simulink model "power_3phlinereclose"  (Simulink 6.0)
settings: Solver=FixedStepDiscrete  StartTime=0.0  StopTime=0.7  FixedStep=50e-6  RelTol=1e-4
undefined symbols (not defined in the file or in its folder): D1, Delta, rvar
libraries: powerlib x24, powerlib_extras x2
settings Model: Creator=sybille  LastModifiedBy=batserve  ExtModeTrigMode=oneshot  ExtModeArmWhenConnect=off  ExtModeAutoUpdateStatusClock=off
settings DataIOCC: LimitDataPoints=off  SignalLoggingName=sigsOut
settings OptimizationCC: BlockReduction=off  BooleanDataType=off
settings DebuggingCC: CheckExecutionContextPreStartOutputMsg=on  CheckExecutionContextRuntimeOutputMsg=on  SolverPrmCheckMsg=none
settings HardwareCC: TargetUnknown=on

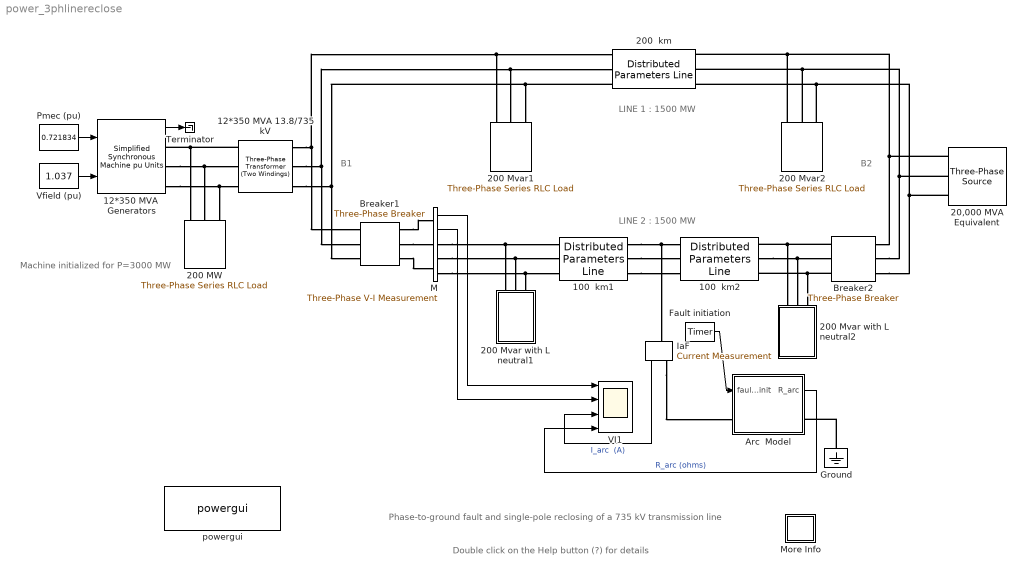
== system power_3phlinereclose ==
  note: Machine initialized
      |  for P=3000 MW
  note: Phase-to-ground fault and single-pole reclosing
      | of  a 735 kV transmission line
  note: Double click on the Help button (?) for details
  note: LINE 1 : 1500 MW
  note: LINE 2 : 1500 MW
  note: B1
  note: B2
  " Breaker1" : powerlib/Elements/Three-Phase Breaker  InitialState=closed  SwitchA=on  SwitchB=off  SwitchC=off  SwitchTimes="[4/60  34/60]"  External=off  BreakerResistance=0.001  SnubberResistance=1e5  SnubberCapacitance=inf  Measurements=None
      settings: AttributesFormatString=\n
  " Breaker2" : powerlib/Elements/Three-Phase Breaker  InitialState=closed  SwitchA=on  SwitchB=off  SwitchC=off  SwitchTimes="[4/60  34/60]"  External=off  BreakerResistance=0.001  SnubberResistance=1e5  SnubberCapacitance=inf  Measurements=None
      settings: AttributesFormatString=\n
  100  km1 : powerlib/Elements/Distributed Parameters Line  Phases=3  Frequency=60  Resistance=[0.01165 0.2676]  Inductance="[0.8679e-3  3.008e-3]"  Capacitance="[13.41e-9  8.57e-9]"  Length=100  x1=[0 4.02705178345773e-008 472803.943791492 -555536.540470784;0.000101545182061977 3.40498179648926e-008 493719.170547751 -537034.187151238;0.000203090364123953 2.77792247481943e-008 513910.94844655 -517744.915291176;0.00030463554618593 2.14679265121164e-008 533349.690387524 -497696.989544924;0.000406180728247907 1.51251712295358e-008 552006.912697188 -476919.786225657;0.000507725910309884 8.76025296747684e-009 569855.276866184 -455443.750260167]  x2=[0 2.22321217810247e-008 426110.546159933 -596874.196271499;0.000101545182061977 1.8422129253629e-008 448642.075203804 -580128.633772847;0.000203090364123953 1.45851426997592e-008 470516.207054946 -562533.006252784;0.00030463554618593 1.0726784472575e-008 491700.889452397 -544113.096661183;0.000406180728247907 6.8527082412422e-009 512165.080388495 -524895.895772037;0.000507725910309884 2.96859070658684e-009 531878.79359486 -504909.562633762]  x3=[0 -4.58387424712223e-010 398.802996869194 -914.417744018894;0.000101545182061977 -4.6900146555621e-010 433.507996432241 -898.484331192913;0.000203090364123953 -4.78928276503843e-010 467.577774834296 -881.234365351327;0.00030463554618593 -4.88153311755674e-010 500.962409480231 -862.69312294444;0.000406180728247907 -4.96663053827248e-010 533.612981719056 -842.88777253575;0.000507725910309884 -5.04445033356331e-010 565.481648524631 -821.847334991732]  x4=[0 5.9976805423792e-010 2831.47677973377 -3826.92877538475;0.000101545182061977 5.94374114547943e-010 2975.86707537689 -3715.75790695924;0.000203090364123953 5.88109235871343e-010 3115.89681999411 -3599.14232224004;0.00030463554618593 5.80982598162212e-010 3251.36082738892 -3477.25289855288;0.000406180728247907 5.73004644113919e-010 3382.06060155949 -3350.26824100279;0.000507725910309884 5.64187063857384e-010 3507.80462755576 -3218.3744207632]  x5=0.000507725910309884  Measurements=None
      settings: AttributesFormatString=\n
  100  km2 : powerlib/Elements/Distributed Parameters Line  Phases=3  Frequency=60  Resistance=[0.01165 0.2676]  Inductance="[0.8679e-3  3.008e-3]"  Capacitance="[13.41e-9  8.57e-9]"  Length=100  x1=[0 2.22321217810247e-008 426110.546159933 -596874.196271499;0.000101545182061977 1.8422129253629e-008 448642.075203804 -580128.633772847;0.000203090364123953 1.45851426997592e-008 470516.207054946 -562533.006252784;0.00030463554618593 1.0726784472575e-008 491700.889452397 -544113.096661183;0.000406180728247907 6.8527082412422e-009 512165.080388495 -524895.895772037;0.000507725910309884 2.96859070658684e-009 531878.79359486 -504909.562633762]  x2=[0 4.59735852839934e-009 372729.13846345 -628102.297137415;0.000101545182061977 3.36982514336241e-009 396494.954357377 -613376.898276943;0.000203090364123953 2.13735393882152e-009 419679.784462561 -597752.715567833;0.00030463554618593 9.01750860216852e-010 442249.655946163 -581252.643193266;0.000406180728247907 -3.3517355786267e-010 464171.497076899 -563900.858781373;0.000507725910309884 -1.57160684466362e-009 485413.185685194 -545722.787977656]  x3=[0 -5.35956762016625e-010 506.939672451892 -849.356884933018;0.000101545182061977 -5.42195113669513e-010 539.075463597358 -829.332546268725;0.000203090364123953 -5.47638984453713e-010 570.421345111015 -808.09298300137;0.00030463554618593 -5.52280397441583e-010 600.931385735744 -785.669317555797;0.000406180728247907 -5.56112551550395e-010 630.560878975732 -762.094407426942;0.000507725910309884 -5.59129831507993e-010 659.266408605095 -737.402797033607]  x4=[0 5.99099720181025e-010 2312.99164112511 -4150.97769376106;0.000101545182061977 5.97237056827686e-010 2470.16390621821 -4059.41308469481;0.000203090364123953 5.94499259405894e-010 2623.71662934839 -3961.90019990165;0.00030463554618593 5.90890339622171e-010 2773.42480903965 -3858.58192543766;0.000406180728247907 5.86415585642443e-010 2919.06907724226 -3749.60965402176;0.000507725910309884 5.81081554343263e-010 3060.43602077378 -3635.14306319931]  x5=0.000507725910309884  Measurements=None
      settings: AttributesFormatString=\n
  12*350 MVA 13.8/735 kV : powerlib/Elements/Three-Phase Transformer (Two Windings)  NominalPower=[ 12*350e6 , 60 ]  Winding1Connection=Delta (D1)  Winding1=[ 13.8e3 , 0.002 , 0.08 ]  Winding2Connection=Yg  Winding2=[ 735e3 , 0.002 , 0.08 ]  SetSaturation=off  Rm=500  Lm=500  Saturation=[ 0,0 ; 0.0024,1.2 ; 1.0,1.52 ]  Hysteresis=off  DataFile='hysteresis'  SetInitialFlux=off  InitialFluxes=[ 0.8 , -0.8 , 0.7 ]  Measurements=None  TransfoNumber=0
  12*350 MVA  Generators : powerlib/Machines/Simplified Synchronous Machine pu Units  ConnectionType=3-wire Y  NominalParameters=[ 12*350e6,13.8e3,60 ]  Mechanical=[ inf,0,2 ]  InternalRL=[ 0.22/15, 0.22 ]  InitialConditions=[0 2.57592 0.717405 0.717405 0.717405 -11.4303 -131.43 108.57]  Units=0  LoadFlowParameters=[1 3000000000 0 0 0]
      settings: AttributesFormatString=\n
  20,000 MVA Equivalent : powerlib/Electrical Sources/Three-Phase Source  Orientation=left  Voltage=735e3  PhaseAngle=0  Frequency=60  InternalConnection=Yg  SpecifyImpedance=on  Resistance=735^2/20000/10  Inductance=735^2/20000/377  ShortCircuitLevel=20000e6  BaseVoltage=735e3  XRratio=10
  200  km : powerlib/Elements/Distributed Parameters Line  Phases=3  Frequency=60  Resistance=[0.01165 0.2676]  Inductance="[0.8679e-3  3.008e-3]"  Capacitance="[13.41e-9  8.57e-9]"  Length=200  x1=[0 7.02850624185661e-008 397648.481541654 -611590.683160231;0.000203090364123953 5.84450393918789e-008 443263.140154233 -579383.379701848;0.000406180728247907 4.62625827673498e-008 486280.688841777 -543781.428257846;0.00060927109237186 3.38090704154687e-008 526449.08475992 -504993.423166597;0.000812361456495814 2.11574683413028e-008 563532.978450831 -463246.626078958;0.00101545182061977 8.38190317153931e-009 597315.092772245 -418785.634416262]  x2=[0 1.07284970616671e-008 289091.132559122 -670718.411670409;0.000203090364123953 8.34931711874698e-009 339546.435190599 -646641.332353954;0.000406180728247907 5.92121793939131e-009 388012.311368668 -618775.53597519;0.00060927109237186 3.45842592752685e-009 434204.796114864 -587284.290195669;0.000812361456495814 9.75370754826919e-010 477853.244411074 -552352.104440056;0.00101545182061977 -1.51339918375015e-009 518701.916927735 -514183.648842435]  x3=[0 -3.94575629964779e-010 275.972756440155 -952.973890092729;0.000203090364123953 -4.20081661821716e-010 348.056371840659 -929.072582426811;0.000406180728247907 -4.43126405666159e-010 418.100700470185 -899.727773133261;0.00060927109237186 -4.63574840722552e-010 485.69534767915 -865.111395514356;0.000812361456495814 -4.81307158171201e-010 550.444271673768 -825.426269362086;0.00101545182061977 -4.96219463116572e-010 611.968103952785 -780.904912622723]  x4=[0 5.79618896597322e-010 1755.99549575464 -4400.33732412217;0.000203090364123953 5.84376073526628e-010 2087.4253958724 -4253.13324126328;0.000406180728247907 5.85709349925921e-010 2406.62492372979 -4081.00975150415;0.00060927109237186 5.83610914034972e-010 2711.72386683501 -3884.97533848145;0.000812361456495814 5.78093060737307e-010 3000.93462901443 -3666.17858161356;0.00101545182061977 5.69188119523618e-010 3272.56270406429 -3425.90142649296]  x5=0.00101545182061977  Measurements=None
      settings: AttributesFormatString=\n
  200 MW : powerlib/Elements/Three-Phase Series RLC Load  Orientation=down  PhysicalDomain=powersysdomain  SubClassName=unknown  LeftPortType=p1  RightPortType=p1  LConnTagsString=A|B|C  Configuration=Y (grounded)  NominalVoltage=13.8e3  NominalFrequency=60  ActivePower=200e6  InductivePower=0  CapacitivePower=0  Measurements=None
  200 Mvar with L neutral1 : Subsystem  Orientation=down
  200 Mvar with L neutral2 : Subsystem  Orientation=down
  200 Mvar1 : powerlib/Elements/Three-Phase Series RLC Load  Orientation=down  PhysicalDomain=powersysdomain  SubClassName=unknown  LeftPortType=p1  RightPortType=p1  LConnTagsString=A|B|C  Configuration=Y (grounded)  NominalVoltage=735e3  NominalFrequency=60  ActivePower=200e6/250  InductivePower=200e6  CapacitivePower=0  Measurements=None
  200 Mvar2 : powerlib/Elements/Three-Phase Series RLC Load  Orientation=down  PhysicalDomain=powersysdomain  SubClassName=unknown  LeftPortType=p1  RightPortType=p1  LConnTagsString=A|B|C  Configuration=Y (grounded)  NominalVoltage=735e3  NominalFrequency=60  ActivePower=200e6/250  InductivePower=200e6  CapacitivePower=0  Measurements=None
  Arc  Model : Subsystem  mask(Arc model){Rarc_var=on, Rarc_fixed=0.1, Rparam=[56.54 0.006375], I0=50, Ts=50e-6}
      mask prompts: Rarc_var "Variable arc resistance :"; Rarc_fixed "Arc resistance for fixed arc resistance :"; Rparam "Arc parameters for variable arc resistance [Ro k] : :"; I0 "Current threshold for arc extinction Io (A rms) :"; Ts "Sample time (s) :"
      mask help:
      | This block implements a variable or fixed arc resistance model.
      |
      | Input 1, output 1:  Connection terminals of the arc
      |                              resistance.
      | Input 2 :    Control signal for the fault initiation
      | Use a short pulse of 1 cycle. Once fault current starts flowing, it is sustained by the arc ionized path.
      | Output 2:  Arc resitance
      |
      | If you check the 'Variable arc resistance' box, the mean arc resistance will be a function of the arc current, according to equation. Otherwise, the resistance will be kept constant.
      |
      |        Rarc= Ro*exp(-k*i)
      |
      | where:   i = rms value of the arc current (A)
      |              Ro, k = arc parameters
      |
      | The arc extinguishes at the next zero current crossing after its  rms value has fallen  below  the specified threshold current Io.
      mask init:
      | if strcmp(Rarc_var,'on'), rvar=1; else, rvar=0; end
      | R0=Rparam(1);
      | k=Rparam(2);
  Fault initiation : powerlib_extras/Control  Blocks/Timer  t=[ 1/60 2/60 ]  e="[1 0  ]"
  Ground : powerlib/Elements/Ground  Orientation=down  PhysicalDomain=powersysdomain  SubClassName=unknown  LeftPortType=p1  RightPortType=p1  LConnTagsString=a
  IaF : powerlib/Measurements/Current Measurement  Tag=PoWeRsYsTeMmEaSuReMeNt  Orientation=down  PhasorSimulation=off  OutputType=Magnitude  PSBequivalent=0
  M : powerlib/Measurements/Three-Phase V-I Measurement  VoltageMeasurement=phase-to-ground  SetLabelV=off  LabelV=V1  Vpu=on  Vbase=735e3  CurrentMeasurement=yes  SetLabelI=off  LabelI=I1  Ipu=on  Pbase=100e6  OutputType=Magnitude  PhasorSimulation=off  PSBequivalent=0
  More Info : Subsystem
      mask Display: disp('?')
  Pmec (pu) : Constant  Value=0.721834
  Terminator : Terminator
  VI1 : Scope  NumInputPorts=4
      settings: TimeRange=0.7000000000000001  YMin=-2~-100~-50000~0  YMax=2~100~50000~100  DataFormat=Array
  Vfield (pu) : Constant  Value=1.037
  powergui : powerlib/powergui  Priority=2  Frange=logspace(0,3,50)  Ylog=off  Xlog=off  save=off  variable=ZData  ZoomFFT=on  StartTime=0.0  cycles=1  DisplayStyle=off  fundamental=60  FreqAxis=off  MaxFrequency=1000  frequencyindice=60  frequencyindicesteady=1  RmsSteady=1  display=off  Ts=50e-6  methode=off  frequency=60  echomessages=on
  wires:
  Fault initiation/1 -> Arc  Model/1(fault_init)
  Arc  Model/1(R_arc) -> VI1/4  "R_arc (ohms)"
  Vfield (pu)/1 -> 12*350 MVA  Generators/2
  Pmec (pu)/1 -> 12*350 MVA  Generators/1
  M/1 -> VI1/1
  IaF/1 -> VI1/3  "I_arc  (A)"
  M/2 -> VI1/2
  12*350 MVA  Generators/1 -> Terminator/1
  connections:
  " Breaker1"/RConn1 -- M/LConn1
  " Breaker1"/RConn2 -- M/LConn2
  " Breaker1"/RConn3 -- M/LConn3
  " Breaker2"/LConn1 -- 100  km2/RConn1 -- 200 Mvar with L neutral2/LConn1
  100  km2/RConn2 -- " Breaker2"/LConn2 -- 200 Mvar with L neutral2/LConn2
  " Breaker2"/LConn3 -- 100  km2/RConn3 -- 200 Mvar with L neutral2/LConn3
  100  km1/RConn1 -- 100  km2/LConn1 -- IaF/LConn1
  " Breaker2"/RConn1 -- 200 Mvar2/LConn1 -- 200  km/RConn1 -- 20,000 MVA Equivalent/RConn1
  " Breaker2"/RConn2 -- 200 Mvar2/LConn2 -- 200  km/RConn2 -- 20,000 MVA Equivalent/RConn2
  " Breaker2"/RConn3 -- 200 Mvar2/LConn3 -- 200  km/RConn3 -- 20,000 MVA Equivalent/RConn3
  M/RConn1 -- 100  km1/LConn1 -- 200 Mvar with L neutral1/LConn1
  M/RConn2 -- 100  km1/LConn2 -- 200 Mvar with L neutral1/LConn2
  M/RConn3 -- 100  km1/LConn3 -- 200 Mvar with L neutral1/LConn3
  100  km1/RConn3 -- 100  km2/LConn3
  100  km1/RConn2 -- 100  km2/LConn2
  12*350 MVA  Generators/RConn2 -- 12*350 MVA 13.8/735 kV/LConn2 -- 200 MW/LConn2
  12*350 MVA 13.8/735 kV/LConn1 -- 12*350 MVA  Generators/RConn1 -- 200 MW/LConn1
  12*350 MVA  Generators/RConn3 -- 12*350 MVA 13.8/735 kV/LConn3 -- 200 MW/LConn3
  12*350 MVA 13.8/735 kV/RConn1 -- " Breaker1"/LConn1 -- 200  km/LConn1 -- 200 Mvar1/LConn1
  12*350 MVA 13.8/735 kV/RConn2 -- " Breaker1"/LConn2 -- 200  km/LConn2 -- 200 Mvar1/LConn2
  200  km/LConn3 -- 12*350 MVA 13.8/735 kV/RConn3 -- " Breaker1"/LConn3 -- 200 Mvar1/LConn3
  IaF/RConn1 -- Arc  Model/LConn1
  Ground/LConn1 -- Arc  Model/RConn1

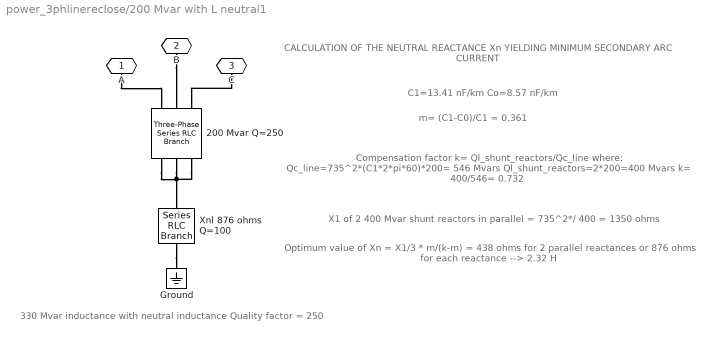
== system power_3phlinereclose/200 Mvar with L neutral1 ==
  note: CALCULATION OF THE NEUTRAL REACTANCE Xn
      | YIELDING MINIMUM SECONDARY ARC CURRENT
  note: X1 of 2 400 Mvar shunt reactors in parallel = 735^2*/ 400 = 1350 ohms
  note: Optimum value of Xn = X1/3 * m/(k-m) = 438 ohms for 2 parallel reactances
      | or 876 ohms for each reactance --> 2.32 H
  note: Compensation factor k= Ql_shunt_reactors/Qc_line
      | where:
      |  Qc_line=735^2*(C1*2*pi*60)*200= 546 Mvars
      |  Ql_shunt_reactors=2*200=400 Mvars
      | k= 400/546= 0.732
  note: m= (C1-C0)/C1 = 0.361
  note: C1=13.41 nF/km Co=8.57 nF/km
  note: 330 Mvar inductance
      | with neutral inductance
      | Quality factor = 250
  200 Mvar Q=250 : powerlib/Elements/Three-Phase Series RLC Branch  Orientation=down  PhysicalDomain=powersysdomain  SubClassName=unknown  LeftPortType=p1  RightPortType=p1  LConnTagsString=A|B|C  RConnTagsString=A|B|C  Resistance=735^2/200/250  Inductance=735^2/200/377  Capacitance=inf  Measurements=None
  Ground : powerlib/Elements/Ground  Orientation=down  PhysicalDomain=powersysdomain  SubClassName=unknown  LeftPortType=p1  RightPortType=p1  LConnTagsString=a
  Xnl 876 ohms Q=100 : powerlib/Elements/Series RLC Branch  Orientation=down  PhysicalDomain=powersysdomain  SubClassName=unknown  LeftPortType=p1  RightPortType=p1  LConnTagsString=__new0  RConnTagsString=__new0  Resistance=876/100  Inductance=876/377  Capacitance=inf  Measurements=None
  A : PMIOPort  Orientation=down  Port=1  Side=Left
  B : PMIOPort  Orientation=down  Port=2  Side=Left
  C : PMIOPort  Orientation=down  Port=3  Side=Left
  connections:
  A/RConn1 -- 200 Mvar Q=250/LConn1
  B/RConn1 -- 200 Mvar Q=250/LConn2
  C/RConn1 -- 200 Mvar Q=250/LConn3
  200 Mvar Q=250/RConn3 -- 200 Mvar Q=250/RConn2 -- Xnl 876 ohms Q=100/LConn1 -- 200 Mvar Q=250/RConn1
  Xnl 876 ohms Q=100/RConn1 -- Ground/LConn1

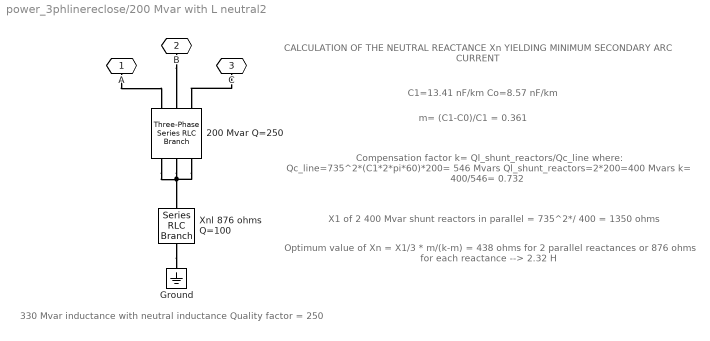
== system power_3phlinereclose/200 Mvar with L neutral2 ==
  note: 330 Mvar inductance
      | with neutral inductance
      | Quality factor = 250
  note: C1=13.41 nF/km Co=8.57 nF/km
  note: m= (C1-C0)/C1 = 0.361
  note: Compensation factor k= Ql_shunt_reactors/Qc_line
      | where:
      |  Qc_line=735^2*(C1*2*pi*60)*200= 546 Mvars
      |  Ql_shunt_reactors=2*200=400 Mvars
      | k= 400/546= 0.732
  note: Optimum value of Xn = X1/3 * m/(k-m) = 438 ohms for 2 parallel reactances
      | or 876 ohms for each reactance --> 2.32 H
  note: X1 of 2 400 Mvar shunt reactors in parallel = 735^2*/ 400 = 1350 ohms
  note: CALCULATION OF THE NEUTRAL REACTANCE Xn
      | YIELDING MINIMUM SECONDARY ARC CURRENT
  200 Mvar Q=250 : powerlib/Elements/Three-Phase Series RLC Branch  Orientation=down  PhysicalDomain=powersysdomain  SubClassName=unknown  LeftPortType=p1  RightPortType=p1  LConnTagsString=A|B|C  RConnTagsString=A|B|C  Resistance=735^2/200/250  Inductance=735^2/200/377  Capacitance=inf  Measurements=None
  Ground : powerlib/Elements/Ground  Orientation=down  PhysicalDomain=powersysdomain  SubClassName=unknown  LeftPortType=p1  RightPortType=p1  LConnTagsString=a
  Xnl 876 ohms Q=100 : powerlib/Elements/Series RLC Branch  Orientation=down  PhysicalDomain=powersysdomain  SubClassName=unknown  LeftPortType=p1  RightPortType=p1  LConnTagsString=__new0  RConnTagsString=__new0  Resistance=876/100  Inductance=876/377  Capacitance=inf  Measurements=None
  A : PMIOPort  Orientation=down  Port=1  Side=Left
  B : PMIOPort  Orientation=down  Port=2  Side=Left
  C : PMIOPort  Orientation=down  Port=3  Side=Left
  connections:
  Xnl 876 ohms Q=100/RConn1 -- Ground/LConn1
  200 Mvar Q=250/RConn3 -- 200 Mvar Q=250/RConn2 -- Xnl 876 ohms Q=100/LConn1 -- 200 Mvar Q=250/RConn1
  C/RConn1 -- 200 Mvar Q=250/LConn3
  B/RConn1 -- 200 Mvar Q=250/LConn2
  A/RConn1 -- 200 Mvar Q=250/LConn1

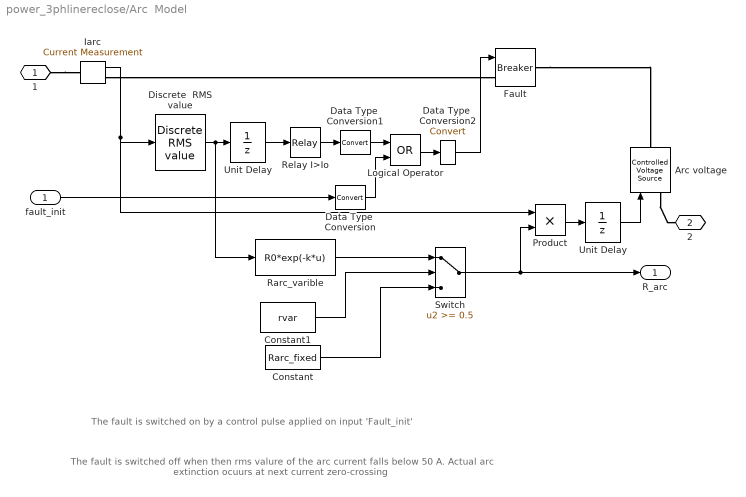
== system power_3phlinereclose/Arc  Model ==
  note: The fault is switched on by a control pulse applied on input 'Fault_init'
  note: The fault is switched off when then rms valure of the arc current falls below  50 A.
      | Actual arc extinction ocuurs at next current zero-crossing
  fault_init : Inport  Port=1  LatchInput=off
  Arc voltage : powerlib/Electrical Sources/Controlled Voltage Source  Description=source block  Orientation=up  Initialize=on  Amplitude=0  Phase=0  Frequency=0  Measurements=None
      settings: AttributesFormatString=\n
  Constant : Constant  Value=Rarc_fixed
  Constant1 : Constant  Value=rvar
  Data Type  Conversion : DataTypeConversion  OutDataTypeMode=boolean  SaturateOnIntegerOverflow=on  RndMeth=Zero
  Data Type  Conversion1 : DataTypeConversion  OutDataTypeMode=boolean  SaturateOnIntegerOverflow=on  RndMeth=Zero
  Data Type  Conversion2 : DataTypeConversion  OutDataTypeMode=double  SaturateOnIntegerOverflow=on  RndMeth=Zero
  Discrete  RMS value : powerlib_extras/Discrete Measurements/Discrete  RMS value  Freq=60  Mag_Init=0  Ts=Ts
  Fault : powerlib/Elements/Breaker  BreakerResistance=.001  InitialState=0  SnubberResistance=inf  SnubberCapacitance=0  SwitchingTimes="[ 4/60  5/60 ]"  External=on  Measurements=None
      settings: AttributesFormatString=\n
  Iarc : powerlib/Measurements/Current Measurement  Tag=PoWeRsYsTeMmEaSuReMeNt  PhasorSimulation=off  OutputType=Magnitude  PSBequivalent=0
  Logical Operator : Logic  Operator=OR
  Product : Product  SaturateOnIntegerOverflow=on  InputSameDT=on
  Rarc_varible : Fcn  Expr=R0*exp(-k*u)
  Relay I>Io : Relay  OnSwitchValue=I0*1.2  OffSwitchValue=I0  ZeroCross=off
  Switch : Switch  Threshold=0.5  ZeroCross=off  InputSameDT=on
  Unit Delay : UnitDelay  SampleTime=Ts
  "Unit Delay " : UnitDelay  SampleTime=Ts
  1 : PMIOPort  Port=1  Side=Left
  2 : PMIOPort  Orientation=left  Port=2  Side=Right
  R_arc : Outport
  wires:
  Discrete  RMS value/1 -> "Unit Delay "/1, Rarc_varible/1
  Rarc_varible/1 -> Switch/1
  Switch/1 -> Product/2, R_arc/1
  Constant/1 -> Switch/3
  Constant1/1 -> Switch/2
  Product/1 -> Unit Delay/1
  "Unit Delay "/1 -> Relay I>Io/1
  fault_init/1 -> Data Type  Conversion/1
  Data Type  Conversion/1 -> Logical Operator/2
  Relay I>Io/1 -> Data Type  Conversion1/1
  Data Type  Conversion1/1 -> Logical Operator/1
  Logical Operator/1 -> Data Type  Conversion2/1
  Iarc/1 -> Product/1, Discrete  RMS value/1
  Unit Delay/1 -> Arc voltage/1
  Data Type  Conversion2/1 -> Fault/1
  connections:
  1/RConn1 -- Iarc/LConn1
  Iarc/RConn1 -- Fault/LConn1
  Arc voltage/LConn1 -- 2/RConn1
  Fault/RConn1 -- Arc voltage/RConn1

== system power_3phlinereclose/More Info ==
  note: Choose Simulation/Start and observe the voltage and current waveforms on the 4-trace oscilloscope.
      |
      | Observe the three phase-to-ground voltages and currents at sending end of line 2 and the current flowing into the fault. The line voltages
      | and currents are measured with the 3-phase measurement bus of the Extras library. It allows to output voltages and currents directly in pu.
      | The machine has been previously initialized to deliver 3000 MW of power at 1 pu voltage (with  the Load Flow option of the Powergui).
      | The line currents flowing into each line are therefore 15pu/100 MVA as observed on trace 2.
      |
      | The fault current (I_arc) is measured in amperes. It reaches 22 kA during the first cycle, then it drops to a very small value after 3 cycles
      |  when the two line breakers open. Use Y-zoom to look at the secondary arc current. It contains a slowly  decaying DC component and a
      |  fundamental component (12 A peak) . As its rms value is below 50 A, the arc extinguishes at the first current zero crossing.
      |
      | Now, open the Arc Model block menu and change the arc model to a fixed resistance (0.1 ohm). Restart the simulation. Notice that the
      | DC component of the arc current prevents arc extinction, so that the line is now  reclosed on a fault.  You can also suppress the neutral
      | reactance in the two shunt reactance blocks and see the impact on the secondary arc current.
  note: Demonstration
  note: Two 735 kV parallel lines, 200 km long, transmit 3000 MW of power from a generation plant (12 generators of 350 MVA) to
      | to an equivalent network having a short circuit level of 20 GVA.
      |
      | The generation plant is simulated with a simplified synchronous machine (subtransient reactance of 0.22 pu).
      | The machine is connected to the transmission network through a 13.8 kV/ 735 kV Wye-Delta transformer.
      |
      | The line models are distributed parameter lines. The lines are assumed to be transposed and their parameters R,L,C /km are specified
      | in positive- and zero-sequence components. Each line is shunt compensated by two shunt reactors of 200 Mvars each, connected at line ends.
      | Applying single pole reclosing at this voltage level is made possible by the use of neutral inductances for the two shunt reactances of line 2.
      | Otherwise, the 'secondary arc current'  which is induced into the fault ( mainly because of the capacitive coupling between the two sound phases
      | and the faulted phase) would be too high to allow arc extinction after opening of  line breakers on the faulted phase.
      | If you open the two shunt reactance blocks of line 2, observe how the optimum neutral inductance is calculated.
  note: This demonstration ilustrates the use of three-phase blocks
      | to study of a single-pole reclosing on  a 735-kV transmission line
  note: Circuit Description
  note: A  phase-to-ground fault is applied at the middle of line 2. In order to apply the fault along the line,
      | this line  is simulated in two sections of 100 km. As soon as the fault is detected by the protection relays (not simulated here) ,
      | an opening command is sent to the two line breakers of the faulted phase. The breaker are kept open during a certain 'dead time' ,
      | usually around 0.5 s, during which the arc normally  extinguishes, then the two breakers are reclosed
      | .
      | When the two line breakers are tripped on the faulted phase, the fault current is interrupted but a small current will continue  to flow through the arc.
      | If this  secondary arc current  is too large (typically above 50 A) , the arc cannot extinguish and the breaker will reclose on the fault..
  note: Fault and line switching
  note: The arc is modelled by a fixed or non-linear resistance R = f(Iarc_rms). The arc extinguishes when its rms current falls below a
      | certain threshold value (typically 50 A) defined in the arc model block. Open the Arc Model block and look at the arc parameters.
      | The mean arc resistance  is programmed as an exponential function of the rms current. The mean arc resistance increases when the rms arc current decreases
      | so that the time for arc current to decay below the threshold value is shortened . (With the specified parameters, Rarc = 0.1ohm and 30 ohms respectively
      | for currents of 1kA and 100A). The Arc Model block  is a masked block. Use 'Look under mask' to see how the arc model is implemented.
      |
      | Open the blocks simulating the two line breakers. See how the line opening/reclosing sequence is programmed.
      | The fault is applied at t = 1 cycle. Then, the opening command is sent to both breakers  at t = 4 cycles (3 cycles detection + opening time).
      | The two breakers are reclosed at t = 34 cycles after a dead time of 30 cycles, during which the arc creating the fault should extinguish.
  note: Arc model
  note: G. Sybille (Hydro-Quebec)
